simulink model "PWC"  (R2014b)
settings: Solver=FixedStepDiscrete  StartTime=0.0  StopTime=10.0  FixedStep=0.1  RelTol=1e-3
settings Model: Creator=z2akhtar  LastModifiedBy=z2akhtar
settings OptimizationCC: ZeroExternalMemoryAtStartup=off  ZeroInternalMemoryAtStartup=off  OptimizeModelRefInitCode=on  LifeSpan=1
settings RTWCC: SystemTargetFile=autosar.tlc  GenCodeOnly=on  TemplateMakefile=ert_default_tmf  Description=AUTOSAR  ProcessScript=autosar_make_rtw_hook
settings CodeAppCC: IgnoreCustomStorageClasses=off
settings STFCustomTargetCC: ParMdlRefBuildCompliant=on  CompOptLevelCompliant=on  IncludeMdlTerminateFcn=off  CombineOutputUpdateFcns=on  SuppressErrorStatus=on  ERTFirstTimeCompliant=on  IncludeFileDelimiter=UseQuote  ERTCustomFileBanners=on  SupportNonFinite=off  SupportComplex=off  SupportContinuousTime=off  SupportNonInlinedSFcns=off  MATLABClassNameForMDSCustomization=Simulink.SoftwareTarget.ERTCustomization  AutosarCompliant=on  GRTInterface=off  SystemTargetFile=autosar.tlc
settings ERTTargetCC: ConcurrentExecutionCompliant=off  IncludeMdlTerminateFcn=off  SuppressErrorStatus=on  IncludeFileDelimiter=UseQuote  SupportNonFinite=off  SupportComplex=off  ModelStepFunctionPrototypeControlCompliant=off  CPPClassGenCompliant=off  AutosarCompliant=on  InlinedParameterPlacement=NonHierarchical  ERTCustomFileTemplate=example_file_process.tlc  GlobalDataDefinition=InSourceFile  GlobalDataReference=InSourceFile  ERTFilePackagingFormat=Compact

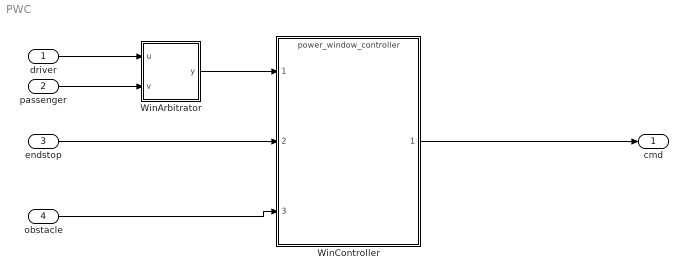
== system PWC ==
  driver : Inport  OutDataTypeStr=uint8
  passenger : Inport  Port=2  OutDataTypeStr=uint8
  endstop : Inport  Port=3  OutDataTypeStr=boolean
  obstacle : Inport  Port=4  OutDataTypeStr=boolean
  WinArbitrator : Truth Table  TreatAsAtomicUnit=on
      settings: RTWSystemCode=Reusable function
  WinController : ModelReference  ModelNameDialog=power_window_controller.slx  SimulationMode=Normal  ModelReferenceVersion=1.53  CopyOfModelName=power_window_controller.slx  DefaultDataLogging=on
  cmd : Outport  OutDataTypeStr=uint8
  wires:
  WinController/1 -> cmd/1
  obstacle/1 -> WinController/3
  driver/1 -> WinArbitrator/1(u)
  passenger/1 -> WinArbitrator/2(v)
  WinArbitrator/1(y) -> WinController/1
  endstop/1 -> WinController/2

== matlab function PWC/WinArbitrator ==
  data: u input uint8; y output uint8; v input uint8
function y = fcn(u, v)

aVarTruthTableCondition_1 = false;
aVarTruthTableCondition_2 = false;
aVarTruthTableCondition_3 = false;
aVarTruthTableCondition_4 = false;


% Example condition 1

aVarTruthTableCondition_1 = logical(u == 0 && v == 0);

% Example condition 2

aVarTruthTableCondition_2 = logical(u == 0 && v == 1);


aVarTruthTableCondition_3 = logical(u == 1 && v == 0);


aVarTruthTableCondition_4 = logical(u == 1 && v == 1);

if (aVarTruthTableCondition_1 && ~aVarTruthTableCondition_2 && aVarTruthTableCondition_3 && aVarTruthTableCondition_4)
    A1();
elseif (~aVarTruthTableCondition_1 && aVarTruthTableCondition_2 && ~aVarTruthTableCondition_3 && ~aVarTruthTableCondition_4)
    A2();
else % Default
    AD();
end

function A1()

% Example action 1 called from D1 & D2 column in condition table

y = u;

function A2()

% Example action 2 called from D3 column in condition table

y = v;

function AD()


y = u;
